simulink model "WATER_TASK3_MAIN"  (R2024b)
settings: Solver=VariableStepAuto  StartTime=0.0  StopTime=300  RelTol=1e-3
settings Model: Creator=Dharmesh  LastModifiedBy=Dharmesh

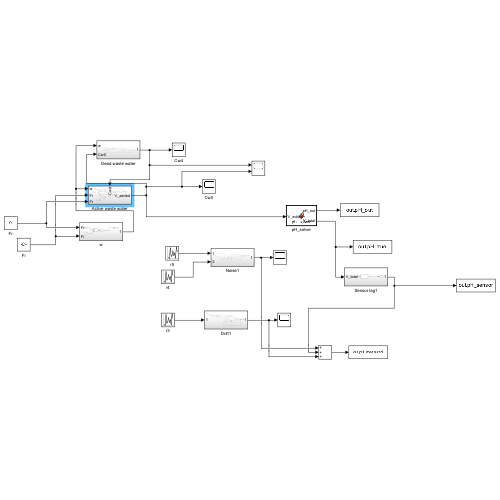
[thumbnail: Simulink's stored preview of the top-level diagram]
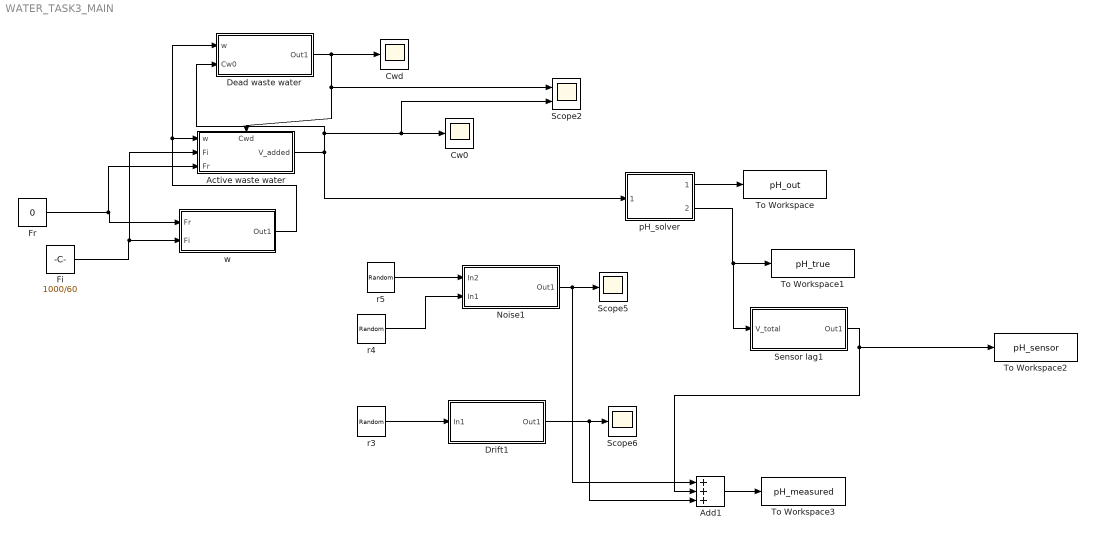
== system WATER_TASK3_MAIN ==
  Active waste water : Subsystem
      settings: PortSchema="{\"entries\":[{\"content\":{\"sides\":[{\"content\":{\"connectorIds\":[\"In1\",\"In2\",\"In3\"]},\"type\":\"ConnectorPlacement.EquallySpacedRectSide\",\"uuid\":\"fdd08be6-e542-434b-bcfd-e03d8eb8934a\"},{\"content\":{\"connectorIds\":[\"Out1\"],\"side\":\"RIGHT\"},\"type\":\"ConnectorPlacement.EquallySpacedRectSide\",\"uuid\":\"3363dfa2-2fb6-4b70-9eec-cac1e7b4f1e0\"},{\"content\":{\"connectorIds\":[\"In4\"],\"side\":\"TOP\"},\"type\":\"ConnectorPlacement.EquallySpacedRectSide\",\"uuid\":\"b10648a6-2485-4102-8fdc-da396d8924bf\"}]},\"type\":\"ConnectorPlacement.EquallySpacedConnector\",\"uuid\":\"036e3afb-3366-4cdb-9c6c-a79e45bd74a4\"}],\"packageUris\":[\"http://schema.mathworks.com/mf0/Connector/R2020b\"],\"version\":\"1.0\"}"
  Add1 : Sum  Inputs=+++
  Cw0 : Scope
  Cwd : Scope
  Dead waste water : Subsystem
  Drift1 : Subsystem
  Fi : Constant  Value=1000/60
  Fr : Constant  Value=0
  Noise1 : Subsystem
  Scope2 : Scope  NumInputPorts=2
  Scope5 : Scope
  Scope6 : Scope
  Sensor lag1 : Subsystem
  To Workspace : ToWorkspace  VariableName=pH_out  SampleTime=-1
  To Workspace1 : ToWorkspace  VariableName=pH_true  SampleTime=0.5
  To Workspace2 : ToWorkspace  VariableName=pH_sensor  SampleTime=0.5
  To Workspace3 : ToWorkspace  VariableName=pH_measured  SampleTime=0.5
  pH_solver : MATLAB Function  TreatAsAtomicUnit=on
  r3 : UniformRandomNumber  Minimum=0  SampleTime=0.1
  r4 : UniformRandomNumber  Minimum=0.000001  SampleTime=0.1
  r5 : UniformRandomNumber  Minimum=0  SampleTime=0.1
  w : Subsystem
  wires:
  Dead waste water/1(Out1) -> Active waste water/4(Cwd), Scope2/1, Cwd/1
  Active waste water/1(V_added) -> pH_solver/1(V_added), Scope2/2, Cw0/1, Dead waste water/2(Cw0)
  Fr/1 -> Active waste water/3(Fr), w/1(Fr)
  Fi/1 -> Active waste water/2(Fi), w/2(Fi)
  w/1(Out1) -> Dead waste water/1(w), Active waste water/1(w)
  pH_solver/2(V_total) -> To Workspace1/1, Sensor lag1/1(V_total)
  pH_solver/1(pH_out) -> To Workspace/1
  Sensor lag1/1(Out1) -> To Workspace2/1, Add1/2
  Add1/1 -> To Workspace3/1
  Noise1/1(Out1) -> Add1/1, Scope5/1
  r3/1 -> Drift1/1(In1)
  r4/1 -> Noise1/2(In1)
  r5/1 -> Noise1/1(In2)
  Drift1/1(Out1) -> Add1/3, Scope6/1

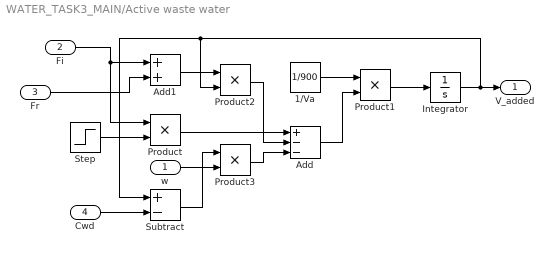
== system WATER_TASK3_MAIN/Active waste water ==
  w : Inport
  Fi : Inport  Port=2
  Fr : Inport  Port=3
  Cwd : Inport  Port=4
  1/Va : Constant  Value=1/900
  Add : Sum  Inputs=+--
  Add1 : Sum
  Integrator : Integrator  InitialCondition=7
  Product{,1..3} (4 alike) : Product
  Step : Step  Time=20  Before=0.1  After=0.2  SampleTime=0
  Subtract : Sum  Inputs=+-
  V_added : Outport
  wires:
  Fi/1 -> Add1/1, Product/1
  Product/1 -> Add/1
  Fr/1 -> Add1/2
  w/1 -> Product3/2
  Step/1 -> Product/2
  Cwd/1 -> Subtract/2
  Add/1 -> Product1/2
  Add1/1 -> Product2/1
  Subtract/1 -> Product3/1
  Product2/1 -> Add/2
  1/Va/1 -> Product1/1
  Product3/1 -> Add/3
  Product1/1 -> Integrator/1
  Integrator/1 -> Subtract/1, Product2/2, V_added/1

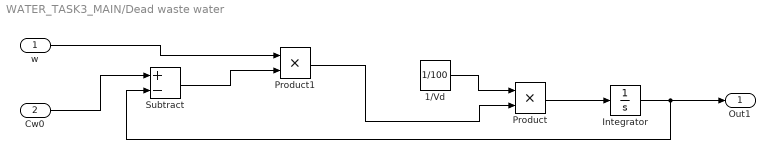
== system WATER_TASK3_MAIN/Dead waste water ==
  w : Inport
  Cw0 : Inport  Port=2
  1/Vd : Constant  Value=1/100
  Integrator : Integrator  InitialCondition=0.001
  Product : Product
  Product1 : Product
  Subtract : Sum  Inputs=+-
  Out1 : Outport
  wires:
  Integrator/1 -> Subtract/2, Out1/1
  Product/1 -> Integrator/1
  1/Vd/1 -> Product/1
  Cw0/1 -> Subtract/1
  Subtract/1 -> Product1/2
  w/1 -> Product1/1
  Product1/1 -> Product/2

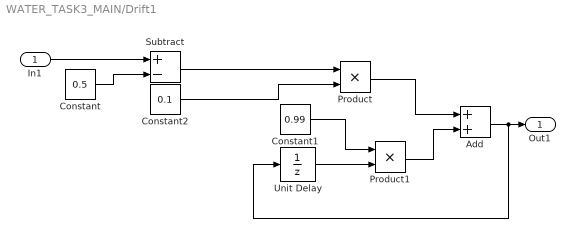
== system WATER_TASK3_MAIN/Drift1 ==
  In1 : Inport
  Add : Sum
  Constant : Constant  Value=0.5
  Constant1 : Constant  Value=0.99
  Constant2 : Constant  Value=0.1
  Product : Product
  Product1 : Product
  Subtract : Sum  Inputs=+-
  Unit Delay : UnitDelay  SampleTime=-1  HasFrameUpgradeWarning=on
  Out1 : Outport
  wires:
  Add/1 -> Unit Delay/1, Out1/1
  In1/1 -> Subtract/1
  Constant/1 -> Subtract/2
  Subtract/1 -> Product/1
  Constant2/1 -> Product/2
  Unit Delay/1 -> Product1/2
  Constant1/1 -> Product1/1
  Product/1 -> Add/1
  Product1/1 -> Add/2

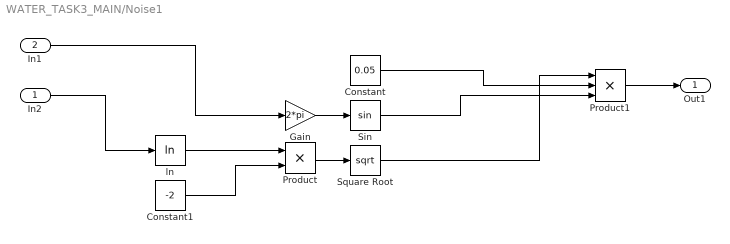
== system WATER_TASK3_MAIN/Noise1 ==
  In2 : Inport
  In1 : Inport  Port=2
  Constant : Constant  Value=0.05
  Constant1 : Constant  Value=-2
  Gain : Gain  Gain=2*pi
  Product : Product
  Product1 : Product  Inputs=3
  Sin : Trigonometry
  Square Root : Sqrt
  ln : Math  Operator=log
  Out1 : Outport
  wires:
  In1/1 -> Gain/1
  In2/1 -> ln/1
  Square Root/1 -> Product1/1
  ln/1 -> Product/1
  Constant/1 -> Product1/2
  Product/1 -> Square Root/1
  Constant1/1 -> Product/2
  Sin/1 -> Product1/3
  Gain/1 -> Sin/1
  Product1/1 -> Out1/1

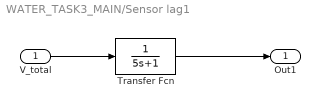
== system WATER_TASK3_MAIN/Sensor lag1 ==
  V_total : Inport
  Transfer Fcn : TransferFcn  Denominator=[5 1]
  Out1 : Outport
  wires:
  V_total/1 -> Transfer Fcn/1
  Transfer Fcn/1 -> Out1/1

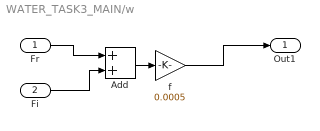
== system WATER_TASK3_MAIN/w ==
  Fr : Inport
  Fi : Inport  Port=2
  Add : Sum
  f : Gain  Gain=0.0005
  Out1 : Outport
  wires:
  Fr/1 -> Add/1
  Fi/1 -> Add/2
  Add/1 -> f/1
  f/1 -> Out1/1

== matlab function WATER_TASK3_MAIN/pH_solver ==
  data: V_added input; pH_out output; V_total output
function [pH_out, V_total] = ph_solver(V_added)
% Computes equilibrium pH for phosphate titration 
% Input : V_added  (L NaOH added)
% Output: pH_out   (equilibrium pH)
%         V_total  (total volume)

% --- Fixed constants ---
V0          = 0.050;           % L initial sample
C_KH2PO4 = 0.100;              
C_titrant   = 0.100;           
Kw          = 1e-14;
Ka1         = 10^(-2.15);
Ka2         = 10^(-7.20);
Ka3         = 10^(-12.35);

% --- Moles and concentrations ---
V_total     = V0 + V_added;
n_P         = C_KH2PO4 * V0;        % total phosphate moles
C_total_P   = n_P / V_total;
n_Na        = C_titrant * V_added;  % moles Na+
C_Na        = n_Na / V_total;
C_K         = (C_KH2PO4 * V0) / V_total; % spectator K+

% --- Bisection for pH between 0 and 14 ---
pH_low = 0; pH_high = 14; tol = 1e-4;
for k = 1:80
    pH_mid = 0.5*(pH_low + pH_high);
    H  = 10^(-pH_mid);
    OH = Kw / H;
    % phosphate fractions α0–α3
    D  = H^3 + H^2*Ka1 + H*Ka1*Ka2 + Ka1*Ka2*Ka3;
    a0 = H^3 / D;                  % H3PO4
    a1 = H^2*Ka1 / D;              % H2PO4−
    a2 = H*Ka1*Ka2 / D;            % HPO4²−
    a3 = Ka1*Ka2*Ka3 / D;          % PO4³−
    % concentrations
    H3PO4 = C_total_P*a0;
    H2PO4 = C_total_P*a1;
    HPO4  = C_total_P*a2;
    PO4   = C_total_P*a3;
    % charge balance residual
    pos = H + C_K + C_Na;
    neg = OH + H2PO4 + 2*HPO4 + 3*PO4;
    res = pos - neg;
    % decide interval
    Hlow = 10^(-pH_low);
    OHlow = Kw / Hlow;
    Dlow = Hlow^3 + Hlow^2*Ka1 + Hlow*Ka1*Ka2 + Ka1*Ka2*Ka3;
    a1low = Hlow^2*Ka1 / Dlow;
    a2low = Hlow*Ka1*Ka2 / Dlow;
    a3low = Ka1*Ka2*Ka3 / Dlow;
    res_low = Hlow + C_K + C_Na - (OHlow + C_total_P*(a1low + 2*a2low + 3*a3low));
    if res_low*res < 0
        pH_high = pH_mid;
    else
        pH_low = pH_mid;
    end
    if abs(pH_high - pH_low) < tol
        break
    end
end
pH_out = pH_mid;
end
